simulink model "PassStCallerForTest"  (R2018b)
settings: Solver=FixedStepDiscrete  StartTime=0.0  StopTime=10.0  RelTol=1e-3
undefined symbols (not defined in the file): PassStFtCtrl_Cal, PassStFtHolderChk_Cal, PassStFtIsPosChk_Cal, PassStFtTrgtPosSelc_Cal, PassStRclCmdSrvCal_Cal
settings Model: Creator=sn2xws  LastModifiedBy=sn2xws
settings DataIOCC: SaveFormat=StructureWithTime
settings OptimizationCC: DefaultParameterBehavior=Inlined  EnhancedBackFolding=on  PassReuseOutputArgsAs=Individual arguments  ZeroExternalMemoryAtStartup=off  ZeroInternalMemoryAtStartup=off  OptimizeBlockOrder=speed  DifferentSizesBufferReuse=on  OptimizationCustomize=off
settings DebuggingCC: ParameterTunabilityLossMsg=error
settings SFSimCC: MATLABDynamicMemAlloc=off
settings RTWCC: SystemTargetFile=autosar.tlc  GenCodeOnly=on  TemplateMakefile=ert_default_tmf  Description=AUTOSAR  GenerateReport=on  IncludeHyperlinkInReport=on  LaunchReport=on  GenerateTraceInfo=on  GenerateTraceReport=on  GenerateTraceReportSl=on  GenerateTraceReportSf=on  GenerateTraceReportEml=on
settings CodeAppCC: ForceParamTrailComments=on  IgnoreCustomStorageClasses=off  OperatorAnnotations=on  SimulinkDataObjDesc=on  SFDataObjDesc=on  InsertBlockDesc=on
settings STFCustomTargetCC: TargetLangStandard=C99 (ISO)  MultiwordLength=256  ParMdlRefBuildCompliant=on  CompOptLevelCompliant=on  IncludeMdlTerminateFcn=off  CombineOutputUpdateFcns=on  SuppressErrorStatus=on  ERTCustomFileBanners=on  SupportNonFinite=off  SupportComplex=off  SupportContinuousTime=off  SupportNonInlinedSFcns=off  RemoveResetFunc=on  MATLABClassNameForMDSCustomization=Simulink.SoftwareTarget.ERTCustomization  AutosarCompliant=on  UseToolchainInfoCompliant=on  LookupTableObjectStructAxisOrder=2,1,3,4,...  LUTObjectStructOrderEvenSpacing=Size,Table,Breakpoints  SystemTargetFile=autosar.tlc
settings ERTTargetCC: TargetLangStandard=C99 (ISO)  ConcurrentExecutionCompliant=off  IncludeMdlTerminateFcn=off  SuppressErrorStatus=on  SupportNonFinite=off  SupportComplex=off  ModelStepFunctionPrototypeControlCompliant=off  CPPClassGenCompliant=off  AutosarCompliant=on  LookupTableObjectStructAxisOrder=2,1,3,4,...  LUTObjectStructOrderEvenSpacing=Size,Table,Breakpoints  InlinedParameterPlacement=NonHierarchical  ERTCustomFileTemplate=example_file_process.tlc  ERTFilePackagingFormat=Compact

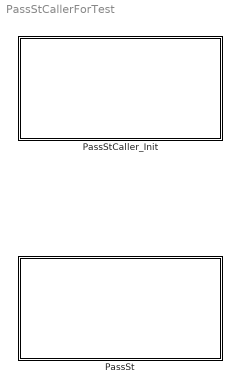
== system PassStCallerForTest ==
  PassSt : Subsystem
  PassStCaller_Init : Subsystem

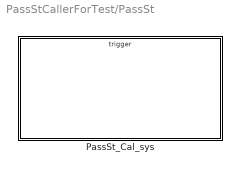
== system PassStCallerForTest/PassSt ==
  PassSt_Cal_sys : Subsystem

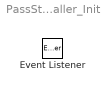
== system PassStCallerForTest/PassStCaller_Init ==
  Event Listener : EventListener  EventName=reset

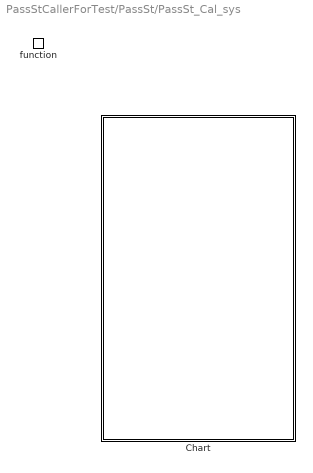
== system PassStCallerForTest/PassSt/PassSt_Cal_sys ==
  function : TriggerPort  TriggerType=function-call  IsSimulinkFunction=on  FunctionName=PassSt_Cal  VariantControl=(inherit)
  Chart : Stateflow chart  TreatAsAtomicUnit=on

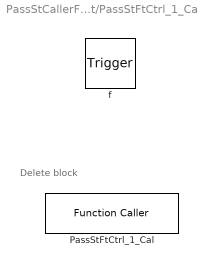
== system PassStCallerForTest/PassSt/PassSt_Cal_sys/Chart/PassStFtCtrl_1_Cal ==
  note: Delete block
  f : TriggerPort  TriggerType=function-call  VariantControl=(inherit)
      settings: CopyFcn=Stateflow.SLINSF.SimulinkMan.removeBlockPreDeleteFcn  PreDeleteFcn=Stateflow.SLINSF.SimulinkMan.unsafePredeleteFcn
  PassStFtCtrl_1_Cal : FunctionCaller  FunctionPrototype=PassStFtCtrl_Cal()

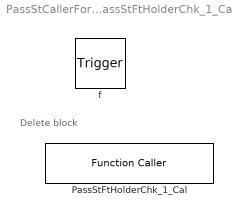
== system PassStCallerForTest/PassSt/PassSt_Cal_sys/Chart/PassStFtHolderChk_1_Cal ==
  note: Delete block
  f : TriggerPort  TriggerType=function-call  VariantControl=(inherit)
      settings: CopyFcn=Stateflow.SLINSF.SimulinkMan.removeBlockPreDeleteFcn  PreDeleteFcn=Stateflow.SLINSF.SimulinkMan.unsafePredeleteFcn
  PassStFtHolderChk_1_Cal : FunctionCaller  FunctionPrototype=PassStFtHolderChk_Cal()

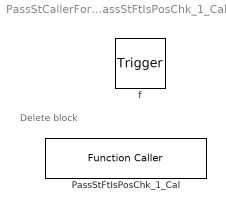
== system PassStCallerForTest/PassSt/PassSt_Cal_sys/Chart/PassStFtIsPosChk_1_Cal ==
  note: Delete block
  f : TriggerPort  TriggerType=function-call  VariantControl=(inherit)
      settings: CopyFcn=Stateflow.SLINSF.SimulinkMan.removeBlockPreDeleteFcn  PreDeleteFcn=Stateflow.SLINSF.SimulinkMan.unsafePredeleteFcn
  PassStFtIsPosChk_1_Cal : FunctionCaller  FunctionPrototype=PassStFtIsPosChk_Cal()

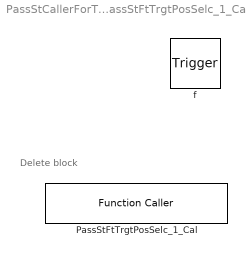
== system PassStCallerForTest/PassSt/PassSt_Cal_sys/Chart/PassStFtTrgtPosSelc_1_Cal ==
  note: Delete block
  f : TriggerPort  TriggerType=function-call  VariantControl=(inherit)
      settings: CopyFcn=Stateflow.SLINSF.SimulinkMan.removeBlockPreDeleteFcn  PreDeleteFcn=Stateflow.SLINSF.SimulinkMan.unsafePredeleteFcn
  PassStFtTrgtPosSelc_1_Cal : FunctionCaller  FunctionPrototype=PassStFtTrgtPosSelc_Cal()

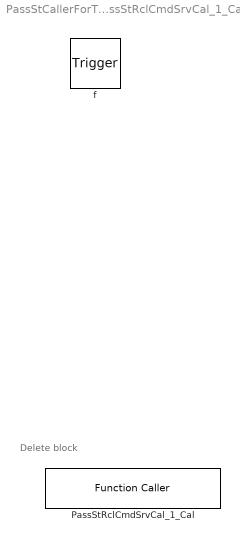
== system PassStCallerForTest/PassSt/PassSt_Cal_sys/Chart/PassStRclCmdSrvCal_1_Cal ==
  note: Delete block
  f : TriggerPort  TriggerType=function-call  VariantControl=(inherit)
      settings: CopyFcn=Stateflow.SLINSF.SimulinkMan.removeBlockPreDeleteFcn  PreDeleteFcn=Stateflow.SLINSF.SimulinkMan.unsafePredeleteFcn
  PassStRclCmdSrvCal_1_Cal : FunctionCaller  FunctionPrototype=PassStRclCmdSrvCal_Cal()

== stateflow chart PassStCallerForTest/PassSt/PassSt_Cal_sys/Chart ==
  state PassStFtTrgtPosSelc_1_Cal [function]
  state PassStFtIsPosChk_1_Cal [function]
  state PassStFtHolderChk_1_Cal [function]
  state PassStFtCtrl_1_Cal [function]
  state PassStRclCmdSrvCal_1_Cal [function]
  (default) -> (junction 1)
  (junction 1) -> (junction 3) : {
      | PassStFtTrgtPosSelc_1_Cal();
      | PassStFtIsPosChk_1_Cal();
      | PassStFtHolderChk_1_Cal();
      | PassStFtCtrl_1_Cal();
      | PassStRclCmdSrvCal_1_Cal();
      | }
